simulink model "User1"  (R2024b)
settings: Solver=FixedStepAuto  StartTime=0.0  StopTime=10.0  RelTol=1e-3
settings Model: Creator=Amin  LastModifiedBy=Amin
settings OptimizationCC: DefaultParameterBehavior=Inlined  EnhancedBackFolding=on  PassReuseOutputArgsAs=Individual arguments  ZeroExternalMemoryAtStartup=off  ZeroInternalMemoryAtStartup=off  OptimizeBlockOrder=speed  DifferentSizesBufferReuse=on  OptimizationCustomize=off  EfficientTunableParamExpr=on
settings DebuggingCC: ParameterTunabilityLossMsg=error
settings SFSimCC: MATLABDynamicMemAlloc=off
settings RTWCC: Description=Embedded Coder  SystemTargetFile=ert.tlc  GenCodeOnly=on  TemplateMakefile=ert_default_tmf  DataTypeReplacement=CDataTypesFixedWidth  TargetLang=C++
settings CodeAppCC: ForceParamTrailComments=on  IgnoreCustomStorageClasses=off  OperatorAnnotations=on  SimulinkDataObjDesc=on  SFDataObjDesc=on  InsertBlockDesc=on
settings ERTTargetCC: TargetLangStandard=C++11 (ISO)  GenerateSampleERTMain=on  SupportAbsoluteTime=off  CodeInterfacePackaging=C++ class  SupportNonFinite=off  SupportComplex=off  RootIOFormat=Structure reference  ERTCustomFileTemplate=example_file_process.tlc  ERTFilePackagingFormat=Compact  MaxIdInt64=INT64_MAX  MinIdInt64=INT64_MIN  MaxIdUint64=UINT64_MAX  MaxIdInt32=INT32_MAX  MinIdInt32=INT32_MIN  MaxIdUint32=UINT32_MAX  MaxIdInt16=INT16_MAX  MinIdInt16=INT16_MIN  MaxIdUint16=UINT16_MAX  MaxIdInt8=INT8_MAX  MinIdInt8=INT8_MIN  MaxIdUint8=UINT8_MAX

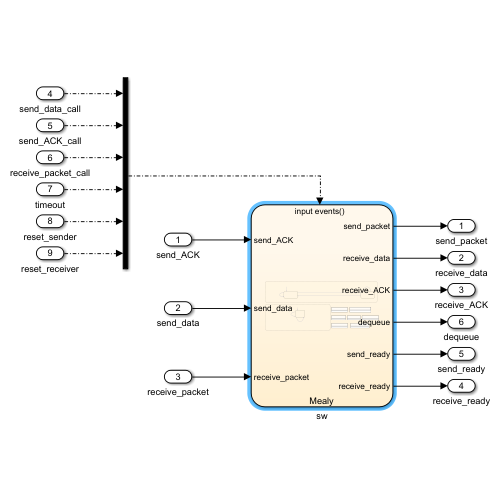
[thumbnail: Simulink's stored preview of the top-level diagram]
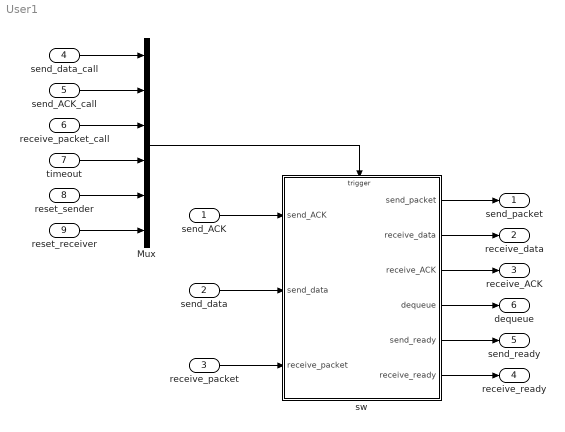
== system User1 ==
  send_ACK : Inport  OutDataTypeStr=uint8
  send_data : Inport  Port=2  OutDataTypeStr=uint8
  receive_packet : Inport  Port=3  OutDataTypeStr=uint16
  send_data_call : Inport  Port=4  OutputFunctionCall=on
  send_ACK_call : Inport  Port=5  OutputFunctionCall=on
  receive_packet_call : Inport  Port=6  OutputFunctionCall=on
  timeout : Inport  Port=7  OutputFunctionCall=on
  reset_sender : Inport  Port=8  OutputFunctionCall=on
  reset_receiver : Inport  Port=9  OutputFunctionCall=on
  Mux : Mux  Inputs=6
  sw : Stateflow chart  TreatAsAtomicUnit=on
  send_packet : Outport  OutDataTypeStr=uint16
  receive_data : Outport  Port=2  OutDataTypeStr=uint8
  receive_ACK : Outport  Port=3  OutDataTypeStr=uint8
  receive_ready : Outport  Port=4  OutDataTypeStr=boolean
  send_ready : Outport  Port=5  OutDataTypeStr=boolean
  dequeue : Outport  Port=6  OutDataTypeStr=boolean
  wires:
  send_ACK/1 -> sw/1(send_ACK)
  sw/1(send_packet) -> send_packet/1
  receive_packet/1 -> sw/3(receive_packet)
  send_ACK_call/1 -> Mux/2
  receive_packet_call/1 -> Mux/3
  Mux/1 -> sw/Trigger
  sw/2(receive_data) -> receive_data/1
  sw/3(receive_ACK) -> receive_ACK/1
  sw/6(receive_ready) -> receive_ready/1
  timeout/1 -> Mux/4
  sw/5(send_ready) -> send_ready/1
  send_data/1 -> sw/2(send_data)
  send_data_call/1 -> Mux/1
  sw/4(dequeue) -> dequeue/1
  reset_sender/1 -> Mux/5
  reset_receiver/1 -> Mux/6

== stateflow chart User1/sw ==
  settings: stateMachineType=MEALY_MACHINE  executeAtInitialization=1
  state send [parallel]
    settings: executionOrder=1
    state Idle
    state Wait_for_ack
    (default) -> Idle
    Wait_for_ack -> Wait_for_ack [order 2] : timeout {send_packet = uint16(calculation(send_data, send_tag));
        | send(send_ready);}
    Idle -> Idle [order 2] : reset_sender{c_ACK = 0; send_tag = 1}
    Idle -> Wait_for_ack [order 1] : send_data_call {send_packet = uint16(calculation(send_data, send_tag)); send(send_ready); dequeue = false}
    Wait_for_ack -> Idle [order 1] : send_ACK_call [checkACK(send_ACK, c_ACK)]{c_ACK = reset_ACK(c_ACK); send_tag = 1-send_tag; dequeue = true;}
  state receive [parallel]
    settings: executionOrder=2
    state state
    (default) -> state
    state -> state [order 2] : reset_receiver{receive_c_ack = 0; receive_tag = 1;}
    state -> state [order 1] : receive_packet_call[check_packet(receive_packet, receive_tag)]
        | {[receive_data, receive_ACK, receive_c_ack] = send_data_ack(receive_packet, receive_c_ack);
        | receive_tag = 1-receive_tag; send(receive_ready);}
  data: value function_input; header function_output; polynomial function_input; p function_input; d function_output; a function_output; c function_input; nc function_output; ca function_input; new_ca function_output; input function_input uint8; output function_output uint16; c_tag function_input; f function_output; ack function_input; check function_input; value function_input; t function_input; header function_output; polynomial function_input; f function_output; p function_input; t function_input; send_packet output uint16; send_ACK input uint8; send_data input uint8 =0; c_ACK local uint8 =0; send_tag local single =1; receive_data output uint8; receive_ACK output uint8; dequeue output boolean =true; receive_c_ack local uint8 =0; receive_tag local single =1; receive_packet input uint16
  events: send_data_call input FUNCTION_CALL_EVENT; send_ACK_call input FUNCTION_CALL_EVENT; send_ready output EITHER_EDGE_EVENT; receive_packet_call input FUNCTION_CALL_EVENT; timeout input FUNCTION_CALL_EVENT; receive_ready output EITHER_EDGE_EVENT; reset_sender input FUNCTION_CALL_EVENT; reset_receiver input FUNCTION_CALL_EVENT
  function header = ack_crc(value, polynomial):
    | function header = ack_crc(value, polynomial)
    |         
    |     % Initialize the CRC register to 0
    |     crc = uint8(0);
    |         
    |     % Loop over each bit in the input byte (MSB first)
    |     for i = 7:-1:-4
    |         % XOR the MSB of the input with the MSB of the CRC register
    |         crc = bitxor(crc, bitand(bitshift(value, -i), 1));  % Shift input and XOR
    |             
    |         % If the MSB of the CRC is 1, perform the polynomial division (XOR)
    |         if bitget(crc, 5)  % Check if MSB (bit 5) of 8-bit crc is set
    |            crc = bitxor(crc, polynomial);  % Perform division by XOR with polynomial
    |         end
    |             
    |         if i ~= -4
    |             % Shift CRC register left by 1 bit
    |             crc = bitshift(crc, 1);
    |         end
    |     end
    |         
    |     
    |     % Final CRC value is the remainder in the lowest 4 bits
    |     header = bitand(crc, 15);  % Mask to get the lower 4 bits as the CRC result
    | end
  function [d, a, nc]= send_data_ack(p, c):
    | function [d, a, nc]= send_data_ack(p, c)
    | 
    |     d = uint8(bitand(p, 0x00FF));
    | 
    |     a = bitor(uint8(c), bitshift(uint8(ack_crc(uint8(c), 19)), 4));
    | 
    |     if c == 15
    |         nc = uint8(0);
    |     else
    |         nc = uint8(c+1);
    |     end
    | 
    | end
  function new_ca = reset_ACK(ca):
    | function new_ca = reset_ACK(ca)
    | 
    |     new_ca = ca + 1;
    | 
    |     if new_ca == 16
    |         new_ca = uint8(0);
    |     end
    | end
  function output = calculation(input, c_tag):
    | function output = calculation(input, c_tag)
    |     
    |     
    |     output = bitor(bitor(uint16(input), bitshift(uint16(c_tag), 8)), bitshift(uint16(crc4(input, c_tag, 19)), 9));
    | 
    | end
  function f = checkACK(ack, check):
    | function f = checkACK(ack, check)
    | 
    |     header = uint8(bitshift(ack, -4));
    |     ack_value = uint8(bitand(ack, 0x0F));
    |     if ack_crc(ack_value, 19) == header && ack_value == check
    |         f = true;
    |     else
    |         f = false;
    |     end
    |     
    | end
  function header = crc4(value, t, polynomial):
    | function header = crc4(value, t, polynomial)
    |         
    |     % Initialize the CRC register to 0
    |     crc = uint16(0);
    |     input = bitor(uint16(value), bitshift(uint16(t), 8));
    |         
    |     % Loop over each bit in the input byte (MSB first)
    |     for i = 8:-1:-4
    |         % XOR the MSB of the input with the MSB of the CRC register
    |         crc = bitxor(crc, bitand(bitshift(input, -i), 1));  % Shift input and XOR
    |             
    |         % If the MSB of the CRC is 1, perform the polynomial division (XOR)
    |         if bitget(crc, 5)  % Check if MSB (bit 5) of 8-bit crc is set
    |            crc = bitxor(crc, polynomial);  % Perform division by XOR with polynomial
    |         end
    |             
    |         if i ~= -4
    |             % Shift CRC register left by 1 bit
    |             crc = bitshift(crc, 1);
    |         end
    |     end
    |         
    |     
    |     % Final CRC value is the remainder in the lowest 4 bits
    |     header = uint8(bitand(crc, 15));  % Mask to get the lower 4 bits as the CRC result
    | end
  function f = check_packet(p, t):
    | function f = check_packet(p, t)
    | 
    |     header = uint8(bitshift(p, -9));
    |     raw_data = uint8(bitand(p, 0x00FF));
    |     checktag = bitget(p, 9);
    |     if crc4(raw_data, receive_tag, 19) == header && checktag == t
    |         f = true;
    |     else
    |         f = false;
    |     end
    |     
    | end
